simulink model "Foguete_Malha_Aberta_ATUAL (1)"  (R2023a)
settings: Solver=VariableStepAuto  StartTime=0.0  StopTime=165  RelTol=1e-3
libraries: simulink x1
settings Model: Creator=pedro
settings OptimizationCC: ReuseModelBlockBuffer=off

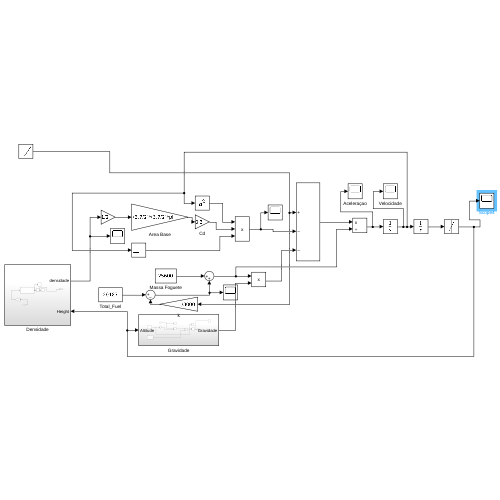
[thumbnail: Simulink's stored preview of the top-level diagram]
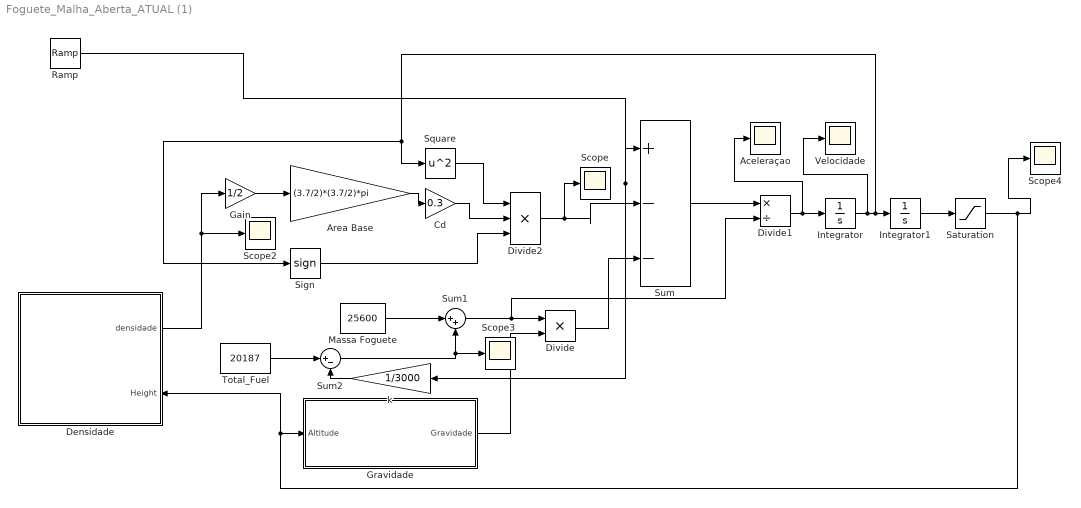
== system Foguete_Malha_Aberta_ATUAL (1) ==
  Aceleraçao : Scope
  Area Base : Gain  Gain=(3.7/2)*(3.7/2)*pi
  Cd : Gain  Gain=0.3
  Densidade : Subsystem
      settings: PortSchema="{\"entries\":[{\"content\":{\"sides\":[{\"content\":{},\"type\":\"ConnectorPlacement.EquallySpacedRectSide\",\"uuid\":\"1cd91c1d-e3da-4072-b1d5-bde77eaa4d77\"},{\"content\":{\"connectorIds\":[\"Out1\",\"In1\"],\"side\":\"RIGHT\"},\"type\":\"ConnectorPlacement.EquallySpacedRectSide\",\"uuid\":\"15adf8d6-6e17-4f5d-b81f-b315088c5251\"},{\"content\":{\"side\":\"TOP\"},\"type\":\"ConnectorPlacement.EquallySpacedRectSide\",\"uuid\":\"e4b32ce3-cb0a-46b5-82b1-bf4ba8b7d084\"}]},\"type\":\"ConnectorPlacement.EquallySpacedConnector\",\"uuid\":\"c32abf6f-6c50-4b1c-8a6c-37657812f68f\"}],\"packageUris\":[\"http://schema.mathworks.com/mf0/Connector/R2020b\"],\"version\":\"1.0\"}"
  Divide : Product  Inputs=**
  Divide1 : Product  Inputs=*/
  Divide2 : Product  Inputs=***
  Gain : Gain  Gain=1/2
  Gravidade : Subsystem
  Integrator : Integrator
  Integrator1 : Integrator  InitialCondition=127*1000
  Massa Foguete : Constant  Value=25600
  Ramp : simulink/Sources/Ramp  slope=15527  start=0  InitialOutput=0
  Saturation : Saturate  UpperLimit=inf  LowerLimit=0
  Scope{,2..4} (4 alike) : Scope
  Sign : Signum
  Square : Math  Operator=square
  Sum : Sum  Inputs=|+--
  Sum1 : Sum  Inputs=|++
  Sum2 : Sum  Inputs=|+-
  Total_Fuel : Constant  Value=20187
  Velocidade : Scope
  k : Gain  Gain=1/3000
  wires:
  Densidade/1(densidade) -> Gain/1, Scope2/1
  Sign/1 -> Divide2/3
  Divide2/1 -> Scope/1, Sum/2
  Square/1 -> Divide2/1
  Saturation/1 -> Scope4/1, Densidade/1(Height), Gravidade/1(Altitude)
  Divide1/1 -> Aceleraçao/1, Integrator/1
  Area Base/1 -> Cd/1
  Sum/1 -> Divide1/1
  Integrator1/1 -> Saturation/1
  Total_Fuel/1 -> Sum2/1
  Sum1/1 -> Divide1/2, Divide/1
  Gravidade/1(Gravidade) -> Divide/2
  Massa Foguete/1 -> Sum1/1
  Gain/1 -> Area Base/1
  Integrator/1 -> Velocidade/1, Square/1, Sign/1, Integrator1/1
  Sum2/1 -> Sum1/2, Scope3/1
  Divide/1 -> Sum/3
  k/1 -> Sum2/2
  Cd/1 -> Divide2/2
  Ramp/1 -> k/1, Sum/1

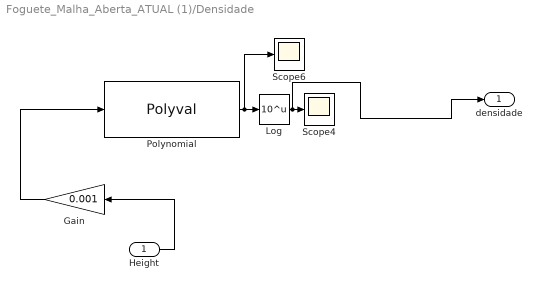
== system Foguete_Malha_Aberta_ATUAL (1)/Densidade ==
  Height : Inport
  Gain : Gain  Gain=0.001
  Log : Math  Operator=10^u
  Polynomial : Polyval  Coefs="[+1.060067e-13, -7.189421e-11, +1.904383e-08,  -2.471283e-06,  +1.621827e-04, -5.009831e-03, -4.336216e-03, 7.001985e-02]"
  Scope4 : Scope
  Scope6 : Scope
  densidade : Outport
  wires:
  Height/1 -> Gain/1
  Log/1 -> densidade/1, Scope4/1
  Gain/1 -> Polynomial/1
  Polynomial/1 -> Log/1, Scope6/1

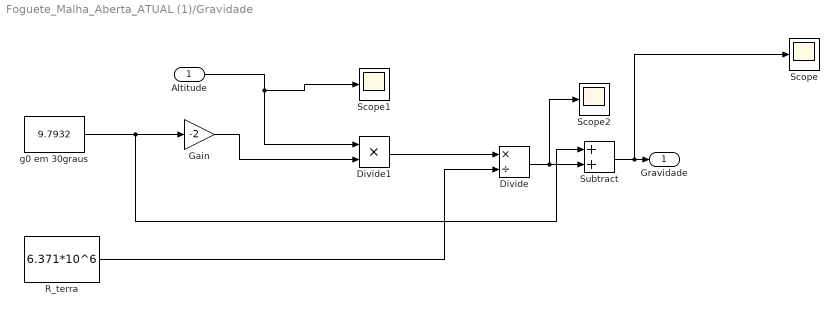
== system Foguete_Malha_Aberta_ATUAL (1)/Gravidade ==
  Altitude : Inport
  Divide : Product  Inputs=*/
  Divide1 : Product  Inputs=**
  Gain : Gain  Gain=-2
  R_terra : Constant  Value=6.371*10^6
  Scope : Scope
  Scope1 : Scope
  Scope2 : Scope
  Subtract : Sum
  g0 em 30graus : Constant  Value=9.7932
  Gravidade : Outport
  wires:
  g0 em 30graus/1 -> Subtract/1, Gain/1
  Gain/1 -> Divide1/2
  Subtract/1 -> Scope/1, Gravidade/1
  Divide/1 -> Scope2/1, Subtract/2
  Divide1/1 -> Divide/1
  R_terra/1 -> Divide/2
  Altitude/1 -> Scope1/1, Divide1/1
